simulink model "Unconnect"  (R2022b)
settings: Solver=FixedStepAuto  StartTime=0.0  StopTime=10.0  FixedStep=0.02  RelTol=1e-3
settings Model: Creator=mganesan  LastModifiedBy=mganesan

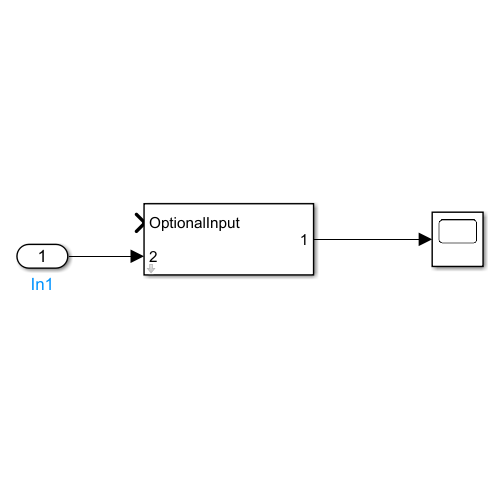
[thumbnail: Simulink's stored preview of the top-level diagram]
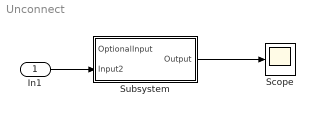
== system Unconnect ==
  In1 : Inport
  Scope : Scope
  Subsystem : Subsystem  mask{Unconnect=0}
      mask init:
      | PL=get_param(gcbh,'LineHandles');
      | if PL.Inport(1) == -1
      |     set_param(gcbh,'MaskValues',{'1'});
      | else
      |     set_param(gcbh,'MaskValues',{'0'});
      | end
  wires:
  Subsystem/1(Output) -> Scope/1
  In1/1 -> Subsystem/2(Input2)

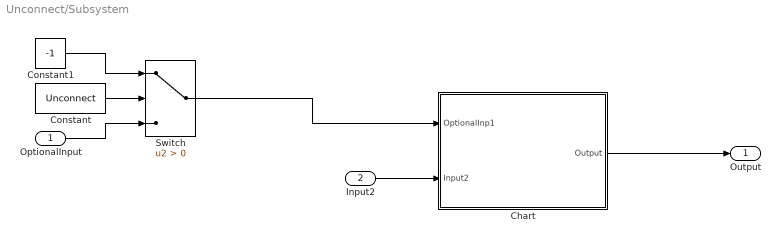
== system Unconnect/Subsystem ==
  OptionalInput : Inport
  Input2 : Inport  Port=2
  Chart : Stateflow chart  TreatAsAtomicUnit=on
  Constant : Constant  Value=Unconnect  OutDataTypeStr=boolean
  Constant1 : Constant  Value=-1
  Switch : Switch  Criteria=u2 > Threshold  SaturateOnIntegerOverflow=off  InputSameDT=off
  Output : Outport
  wires:
  Constant/1 -> Switch/2
  Switch/1 -> Chart/1(OptionalInp1)
  Input2/1 -> Chart/2(Input2)
  Chart/1(Output) -> Output/1
  Constant1/1 -> Switch/1
  OptionalInput/1 -> Switch/3

== stateflow chart Unconnect/Subsystem/Chart ==
  state Init
    en: Output=0;
  state Run1
    en, du: Output=100;
  state Run
    en, du: Output=Output+1;
  (default) -> Init
  Init -> Run1 [order 2] : [OptionalInp1==-1]
  Init -> Run [order 1] : [OptionalInp1==0]
  Run -> Init [order 1] : [OptionalInp1~=0]
  Run -> Run1 [order 2] : [OptionalInp1==-1]
  data: OptionalInp1 input double size=1; Input2 input double size=1; Output output double size=1
